simulink model "case_4_lead_disappears"  (R2025b)
settings: Solver=VariableStepAuto  StartTime=0.0  StopTime=10.0  RelTol=1e-3
settings Model: Creator=sanborkl  LastModifiedBy=admin

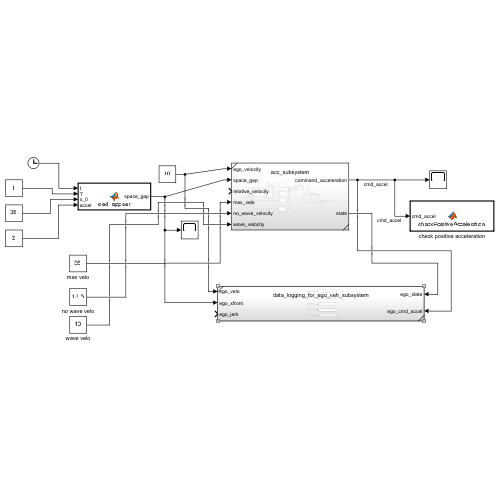
[thumbnail: Simulink's stored preview of the top-level diagram]
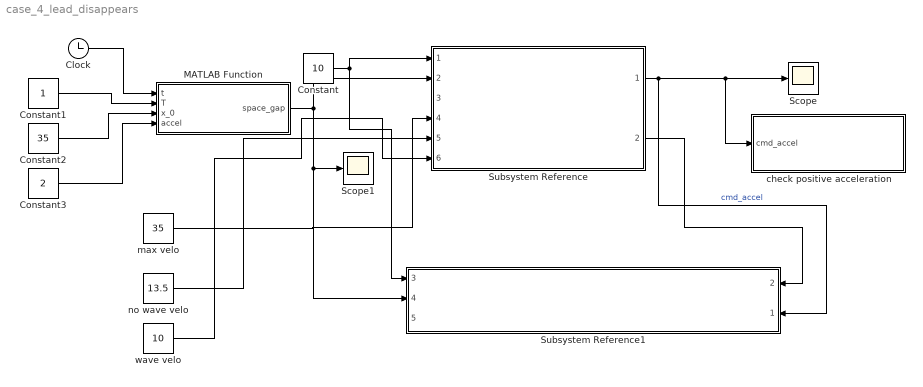
== system case_4_lead_disappears ==
  Clock : Clock
  Constant : Constant  Value=10
  Constant1 : Constant
  Constant2 : Constant  Value=35
  Constant3 : Constant  Value=2
  MATLAB Function : MATLAB Function  TreatAsAtomicUnit=on
  Scope : Scope
      settings: ActiveDisplayYMinimum=-3.5625  ActiveDisplayYMaximum=2.0625
  Scope1 : Scope
      settings: ActiveDisplayYMinimum=-14.374999999999993  ActiveDisplayYMaximum=329.375
  Subsystem Reference : Subsystem  ReferencedSubsystem=acc_subsystem
  Subsystem Reference1 : Subsystem  ReferencedSubsystem=data_logging_for_ego_veh_subsystem
      settings: PortSchema="{\"entries\":[{\"content\":{\"sides\":[{\"content\":{\"connectorIds\":[\"In3\",\"In4\",\"In5\"]},\"type\":\"ConnectorPlacement.EquallySpacedRectSide\",\"uuid\":\"0b96bcaa-a470-46c9-9268-f4bd6b1035a8\"},{\"content\":{\"connectorIds\":[\"In2\",\"In1\"],\"side\":\"RIGHT\"},\"type\":\"ConnectorPlacement.EquallySpacedRectSide\",\"uuid\":\"8e49005a-1e53-4e76-b163-50df0eb9f2cc\"},{\"content\":{\"side\":\"TOP\"},\"type\":\"ConnectorPlacement.EquallySpacedRectSide\",\"uuid\":\"3ff4af65-efca-4a64-9b7f-f479498e89e2\"}]},\"type\":\"ConnectorPlacement.EquallySpacedConnector\",\"uuid\":\"f10caef7-9599-4d5c-a8fd-3eb49f6fcaa8\"}],\"packageUris\":[\"http://schema.mathworks.com/mf0/Connector/R2020b\"],\"version\":\"1.0\"}"
  check positive acceleration : MATLAB Function  TreatAsAtomicUnit=on
  max velo : Constant  Value=35
  no wave velo : Constant  Value=13.5
  wave velo : Constant  Value=10
  wires:
  Constant/1 -> Subsystem Reference1/3, Subsystem Reference/1
  MATLAB Function/1(space_gap) -> Subsystem Reference1/4, Scope1/1, Subsystem Reference/2
  Clock/1 -> MATLAB Function/1(t)
  Constant1/1 -> MATLAB Function/2(T)
  Constant2/1 -> MATLAB Function/3(x_0)
  Constant3/1 -> MATLAB Function/4(accel)
  Subsystem Reference/1 -> Subsystem Reference1/1, Scope/1, check positive acceleration/1(cmd_accel)  "cmd_accel"
  Subsystem Reference/2 -> Subsystem Reference1/2
  max velo/1 -> Subsystem Reference/4
  no wave velo/1 -> Subsystem Reference/5
  wave velo/1 -> Subsystem Reference/6

== matlab function case_4_lead_disappears/MATLAB Function ==
  data: t input; space_gap output; T input; x_0 input; accel input
function space_gap = lead_appear(t, T, x_0, accel)

if (t <= T)
    space_gap = x_0 + accel * t;
else
    space_gap = (x_0 + accel * t) + 255;
end

== matlab function case_4_lead_disappears/check positive acceleration ==
  data: cmd_accel input
function checkPositiveAcceleration(cmd_accel)
%#codegen
coder.extrinsic('disp', 'sprintf');

if cmd_accel < 0
    msg = sprintf('Error: Negative command acceleration: %.3f, should be positive', ...
                  cmd_accel);
    disp(msg);
end
end
